simulink model "Lab_Practice6_1_SML"  (R2024b)
settings: Solver=ode45  StartTime=0.0  StopTime=t_sim  MaxStep=0.0001*Ts  MinStep=0.00001*Ts  RelTol=1e-3
values from neighbouring files (symbols this model uses):
  C = [1 0]    [Lab_Practice6_1.m]
  md = MPCInit(Ad,Bd,Cy,Cz,Dz,Cc,Dc,Hp,Hw,z_blk,Hu,u_blk,du_max,du_min,u_max,u_min,z_max,z_min,Q,R,[],[],h,cmode,'qp_as')    [Lab_Practice6_1.m]
  rho = 1    [Lab_Practice6_1.m]
  Ts = 0.05    [Lab_Practice6_1.m]    (also in Lab_Practice6_3.m = 0.2; Lab_Practice6_4.m = 0.2)
  x0 = [0;0]    [Lab_Practice6_1.m]    (also in Lab_Practice6_3.m = [-0.3;0.4]; Lab_Practice6_4.m = [-0.3;0.4])
libraries: cstblocks x1
settings Model: Creator=filoz  LastModifiedBy=filoz
settings SolverCC: InitialStep=0.00001*Ts

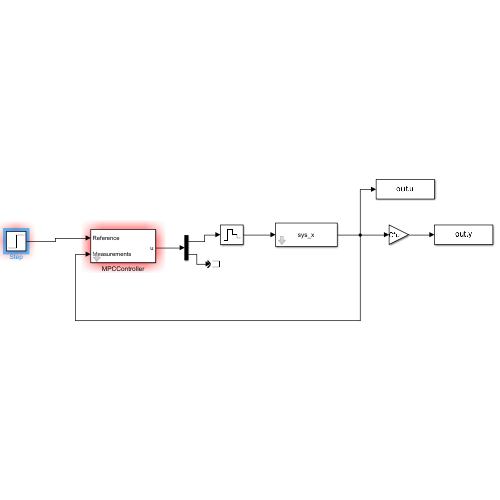
[thumbnail: Simulink's stored preview of the top-level diagram]
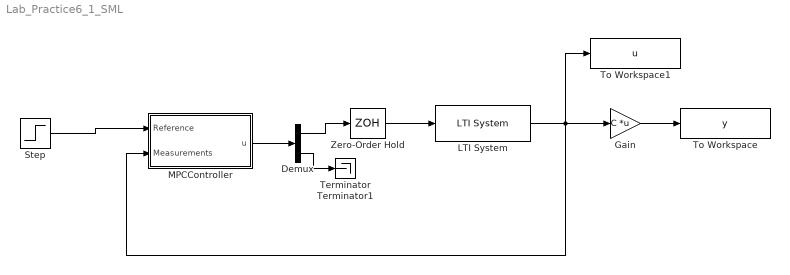
== system Lab_Practice6_1_SML ==
  Demux : Demux  Outputs=2
  Gain : Gain  Gain=C  Multiplication=Matrix(K*u)
  LTI System : cstblocks/LTI System  sys=sys_x  IC=[x0]  PadeOrder=0
  MPCController : Subsystem  mask{md=md}
      mask prompts: md "MPCData"
  Step : Step  Time=0  After=rho  SampleTime=Ts
  Terminator : Terminator
  Terminator1 : Terminator
  To Workspace : ToWorkspace  VariableName=y  SaveFormat=Timeseries  SampleTime=0.01*Ts
  To Workspace1 : ToWorkspace  VariableName=u  SaveFormat=Timeseries  SampleTime=0.01*Ts
  Zero-Order Hold : ZeroOrderHold  SampleTime=Ts
  wires:
  Zero-Order Hold/1 -> LTI System/1
  Demux/2 -> Terminator1/1
  LTI System/1 -> To Workspace1/1, MPCController/2(Measurements), Gain/1
  Gain/1 -> To Workspace/1
  Demux/1 -> Zero-Order Hold/1
  MPCController/1(u) -> Demux/1
  Step/1 -> MPCController/1(Reference)

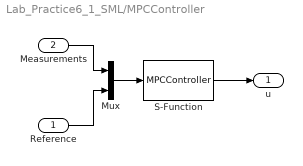
== system Lab_Practice6_1_SML/MPCController ==
  Reference : Inport
  Measurements : Inport  Port=2
  Mux : Mux  Inputs=2
  S-Function : S-Function  FunctionName=MPCController  Parameters=md  SFunctionDeploymentMode=off  EnableBusSupport=off
  u : Outport
  wires:
  Mux/1 -> S-Function/1
  Measurements/1 -> Mux/1
  Reference/1 -> Mux/2
  S-Function/1 -> u/1
